simulink model "a2sw_nl_ged_sub"  (R2020b)
settings: Solver=ode45  StartTime=0.0  StopTime=30.0  MaxStep=0.01  RelTol=1e-3  EnableMultiTasking=on
model workspace (MAT data in the model file):
  c = 0.1
  delta = 0.1
  k = 1
  m = 2
  v0 = 0
  y0 = 2
settings Model: Creator=Reichl  LastModifiedBy=jakob
settings DataIOCC: LimitDataPoints=on  SaveFormat=Array  SignalLoggingSaveFormat=ModelDataLogs  ReturnWorkspaceOutputs=off
settings OptimizationCC: ExpressionDepthLimit=2147483647  LifeSpan=inf
settings DebuggingCC: UnderspecifiedInitializationDetection=Classic  MergeDetectMultiDrivingBlocksExec=none  SolverPrmCheckMsg=warning  FcnCallInpInsideContextMsg=warning  StateNameClashWarn=warning  SFUnexpectedBacktrackingDiag=warning  SFNoUnconditionalDefaultTransitionDiag=warning  SFExecutionAtInitializationDiag=none  ArithmeticOperatorsInVariantConditions=warning
settings HardwareCC: ProdBitPerPointer=32  ProdBitPerSizeT=32  ProdBitPerPtrDiffT=32  ProdLargestAtomicFloat=None  ProdIntDivRoundTo=Undefined  ProdEndianess=Unspecified  ProdWordSize=32  ProdHWDeviceType=32-bit Generic
settings ModelReferenceCC: PropagateSignalLabelsOutOfModel=off
settings SFSimCC: SimUseLocalCustomCode=off  CustomCodeUndefinedFunction=UseInterfaceOnly
settings RTWCC: RTWUseLocalCustomCode=off
settings CodeAppCC: StateflowObjectComments=on
settings GRTTargetCC: TargetLangStandard=C89/C90 (ANSI)  CombineOutputUpdateFcns=off  GRTInterface=on
settings ConfigComp: CovMetricSettings=dw  CovSaveCumulativeToWorkspaceVar=on  CovSaveSingleToWorkspaceVar=on  CovExternalEMLEnable=off  CovSFcnEnable=off

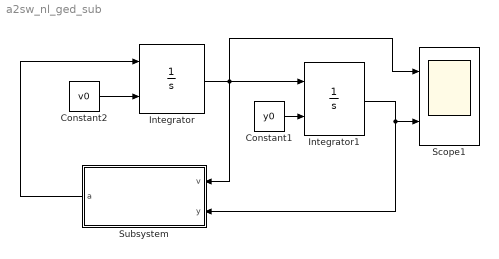
== system a2sw_nl_ged_sub ==
  " Constant2" : Constant  Value=v0
  Constant1 : Constant  Value=y0
  Integrator : Integrator  InitialConditionSource=external
  Integrator1 : Integrator  InitialConditionSource=external  InitialCondition=3
  Scope1 : Scope  NumInputPorts=2
  Subsystem : Subsystem
  wires:
  Integrator/1 -> Scope1/1, Subsystem/1(v), Integrator1/1
  " Constant2"/1 -> Integrator/2
  Constant1/1 -> Integrator1/2
  Subsystem/1(a) -> Integrator/1
  Integrator1/1 -> Subsystem/2(y), Scope1/2

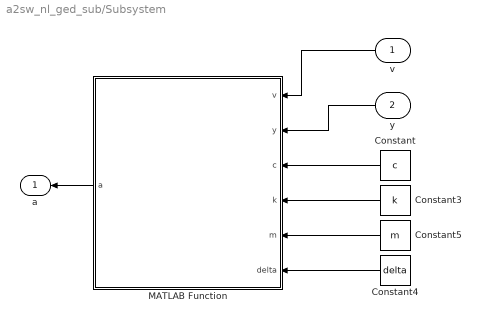
== system a2sw_nl_ged_sub/Subsystem ==
  v : Inport
  y : Inport  Port=2
  Constant : Constant  Value=c
  Constant3 : Constant  Value=k
  Constant4 : Constant  Value=delta
  Constant5 : Constant  Value=m
  MATLAB Function : MATLAB Function  TreatAsAtomicUnit=on
  a : Outport  VectorParamsAs1DForOutWhenUnconnected=off
  wires:
  v/1 -> MATLAB Function/1(v)
  y/1 -> MATLAB Function/2(y)
  MATLAB Function/1(a) -> a/1
  Constant5/1 -> MATLAB Function/5(m)
  Constant/1 -> MATLAB Function/3(c)
  Constant4/1 -> MATLAB Function/6(delta)
  Constant3/1 -> MATLAB Function/4(k)

== matlab function a2sw_nl_ged_sub/Subsystem/MATLAB Function ==
  data: v input; y input; a output; c input; k input; m input; delta input
function a = fcn(v,y,c,k,m,delta)

a= -2*delta*v-k/m*y-c/m*y^3;
